simulink model "AAI"  (R2022a)
settings: Solver=FixedStepAuto  StartTime=0.0  StopTime=10.0  FixedStep=1e-3  RelTol=1e-3  EnableMultiTasking=on
undefined symbols (not defined in the file or in its folder): D0, D10, D11, D12, D2, D4, D5, D6, D7, D8, D9, PTA0, PTA2, PTB23, PTB9, PTC16, PTC2, PTC3, PTC4, PTD0, PTD2, PTD3
libraries: frdmk64flib x11
settings Model: ExtModeTrigDuration=5  Creator=anand  LastModifiedBy=anand
settings OptimizationCC: EnhancedBackFolding=on  PassReuseOutputArgsAs=Individual arguments  ZeroExternalMemoryAtStartup=off  ZeroInternalMemoryAtStartup=off  MaxStackSize=64  OptimizeBlockOrder=speed  DifferentSizesBufferReuse=on  OptimizationCustomize=off  EfficientTunableParamExpr=on
settings DebuggingCC: ParameterTunabilityLossMsg=error
settings HardwareCC: ProdBitPerPointer=32  ProdBitPerSizeT=32  ProdBitPerPtrDiffT=32  ProdLargestAtomicInteger=Long  ProdLargestAtomicFloat=Double  ProdWordSize=32  ProdHWDeviceType=ARM Compatible->ARM Cortex
settings SFSimCC: MATLABDynamicMemAlloc=off
settings RTWCC: SystemTargetFile=ert.tlc  HardwareBoard=NXP FRDM-K64F  TLCOptions="-aInlineSetEventsForThisBaseRateFcn=TLC_FALSE -aSuppressMultiTaskScheduler=TLC_FALSE  -aRateBasedStepFcn=0"  TemplateMakefile=ert_default_tmf  Toolchain=GNU Tools for ARM Embedded Processors
settings CodeAppCC: ForceParamTrailComments=on  IgnoreCustomStorageClasses=off  OperatorAnnotations=on  SimulinkDataObjDesc=on  SFDataObjDesc=on  InsertBlockDesc=on
settings ERTTargetCC: ExtModeTransport=4  ExtModeMexFile=sendToCommService

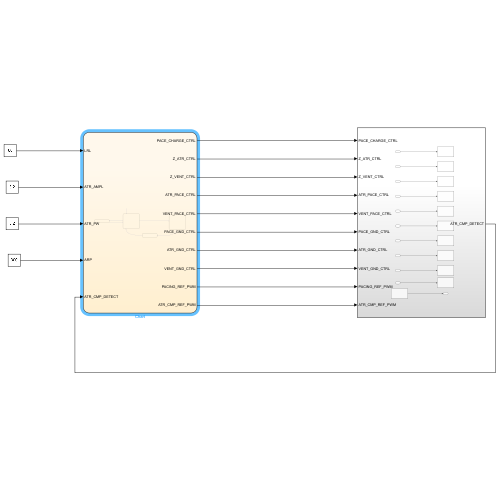
[thumbnail: Simulink's stored preview of the top-level diagram]
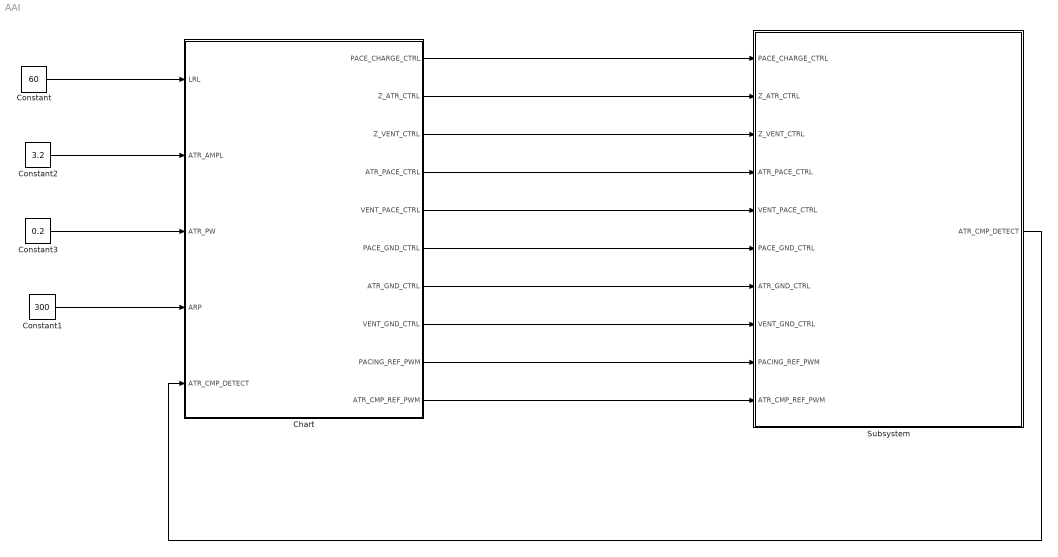
== system AAI ==
  Chart : Stateflow chart  TreatAsAtomicUnit=on
  Constant : Constant  Value=60
  Constant1 : Constant  Value=300
  Constant2 : Constant  Value=3.2
  Constant3 : Constant  Value=0.2
  Subsystem : Subsystem
  wires:
  Subsystem/1(ATR_CMP_DETECT) -> Chart/5(ATR_CMP_DETECT)
  Constant2/1 -> Chart/2(ATR_AMPL)
  Chart/3(Z_VENT_CTRL) -> Subsystem/3(Z_VENT_CTRL)
  Chart/10(ATR_CMP_REF_PWM) -> Subsystem/10(ATR_CMP_REF_PWM)
  Chart/1(PACE_CHARGE_CTRL) -> Subsystem/1(PACE_CHARGE_CTRL)
  Chart/9(PACING_REF_PWM) -> Subsystem/9(PACING_REF_PWM)
  Constant/1 -> Chart/1(LRL)
  Chart/6(PACE_GND_CTRL) -> Subsystem/6(PACE_GND_CTRL)
  Chart/7(ATR_GND_CTRL) -> Subsystem/7(ATR_GND_CTRL)
  Constant1/1 -> Chart/4(ARP)
  Chart/4(ATR_PACE_CTRL) -> Subsystem/4(ATR_PACE_CTRL)
  Constant3/1 -> Chart/3(ATR_PW)
  Chart/8(VENT_GND_CTRL) -> Subsystem/8(VENT_GND_CTRL)
  Chart/2(Z_ATR_CTRL) -> Subsystem/2(Z_ATR_CTRL)
  Chart/5(VENT_PACE_CTRL) -> Subsystem/5(VENT_PACE_CTRL)

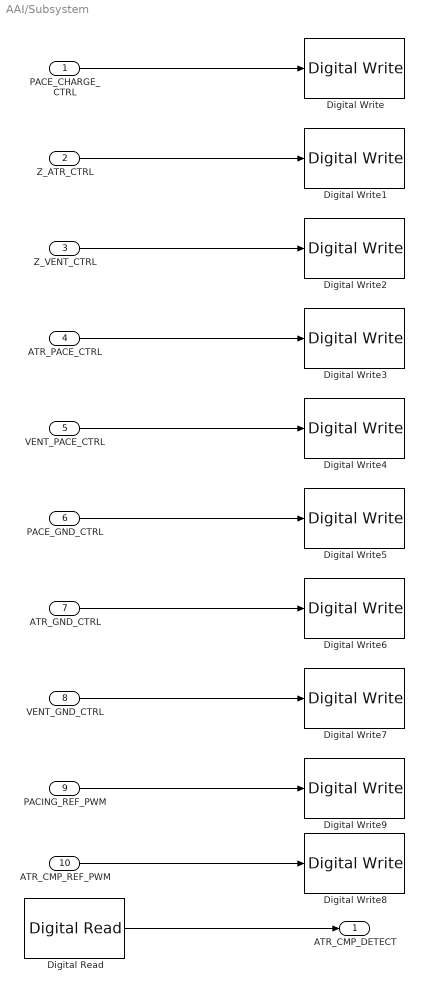
== system AAI/Subsystem ==
  PACE_CHARGE_CTRL : Inport  OutDataTypeStr=boolean
  Z_ATR_CTRL : Inport  Port=2  OutDataTypeStr=boolean
  Z_VENT_CTRL : Inport  Port=3
  ATR_PACE_CTRL : Inport  Port=4
  VENT_PACE_CTRL : Inport  Port=5
  PACE_GND_CTRL : Inport  Port=6
  ATR_GND_CTRL : Inport  Port=7
  VENT_GND_CTRL : Inport  Port=8
  PACING_REF_PWM : Inport  Port=9
  ATR_CMP_REF_PWM : Inport  Port=10
  Digital Read : frdmk64flib/Digital Read  Whichpin=PTC16 (D0)  SampleTime=-1
  Digital Write : frdmk64flib/Digital Write  Whichpin=PTB9 (D2)
  Digital Write1 : frdmk64flib/Digital Write  Whichpin=PTB23 (D4)
  Digital Write2 : frdmk64flib/Digital Write  Whichpin=PTC3 (D7)
  Digital Write3 : frdmk64flib/Digital Write  Whichpin=PTA0 (D8)
  Digital Write4 : frdmk64flib/Digital Write  Whichpin=PTC4 (D9)
  Digital Write5 : frdmk64flib/Digital Write  Whichpin=PTD0 (D10)
  Digital Write6 : frdmk64flib/Digital Write  Whichpin=PTD2 (D11)
  Digital Write7 : frdmk64flib/Digital Write  Whichpin=PTD3 (D12)
  Digital Write8 : frdmk64flib/Digital Write  Whichpin=PTC2 (D6)
  Digital Write9 : frdmk64flib/Digital Write  Whichpin=PTA2 (D5)
  ATR_CMP_DETECT : Outport  OutDataTypeStr=boolean
  wires:
  PACE_CHARGE_CTRL/1 -> Digital Write/1
  Z_ATR_CTRL/1 -> Digital Write1/1
  Z_VENT_CTRL/1 -> Digital Write2/1
  ATR_PACE_CTRL/1 -> Digital Write3/1
  VENT_PACE_CTRL/1 -> Digital Write4/1
  PACE_GND_CTRL/1 -> Digital Write5/1
  ATR_GND_CTRL/1 -> Digital Write6/1
  VENT_GND_CTRL/1 -> Digital Write7/1
  PACING_REF_PWM/1 -> Digital Write9/1
  ATR_CMP_REF_PWM/1 -> Digital Write8/1
  Digital Read/1 -> ATR_CMP_DETECT/1

== stateflow chart AAI/Chart ==
  state CHARGING
    entry:
    %CHARGING C22
    ATR_PACE_CTRL = false;
    VENT_PACE_CTRL = false;
    PACING_REF_PWM = 100*ATR_AMPL/5;
    ATR_CMP_REF_PWM = 100*ATR_AMPL/5;
    PACE_CHARGE_CTRL = true
  state PACE_ATR
    entry:
    PACE_CHARGE_CTRL = false;
    PACE_GND_CTRL = true;
    ATR_PACE_CTRL = true;
    ATR_GND_CTRL = false;
    Z_ATR_CTRL = false;
    Z_VENT_CTRL = false;
    VENT_GND_CTRL = false;
    VENT_PACE_CTRL = false;
  state Atrial_Refractory_Period_Post_Sensing
  state DISCHARGING
    entry:
    %DISCHARGING C21
    PACE_GND_CTRL = true;
    VENT_PACE_CTRL = false;
    Z_ATR_CTRL = false;
    Z_VENT_CTRL = false;
    ATR_PACE_CTRL = false;
    ATR_GND_CTRL = true;
    VENT_GND_CTRL = false;
  (default) -> CHARGING : {delta = 0;}
  CHARGING -> PACE_ATR [order 2] : [after(60000/LRL-delta-ATR_PW, msec)]
  CHARGING -> Atrial_Refractory_Period_Post_Sensing [order 1] : [ATR_CMP_DETECT(1) ==1]
  Atrial_Refractory_Period_Post_Sensing -> CHARGING : [after(ARP,msec)]{delta = ARP}
  DISCHARGING -> CHARGING : [after(ARP,msec)]{delta=ARP;}
  PACE_ATR -> DISCHARGING : [after(ATR_PW,msec)]
  data: LRL input; ATR_AMPL input; ATR_PW input; PACE_CHARGE_CTRL output boolean; Z_ATR_CTRL output; Z_VENT_CTRL output; ATR_PACE_CTRL output; VENT_PACE_CTRL output; PACE_GND_CTRL output; ATR_GND_CTRL output; VENT_GND_CTRL output; PACING_REF_PWM output; ARP input; ATR_CMP_DETECT input boolean size=[1,1]; ATR_CMP_REF_PWM output; delta local double
